simulink model "gearBoxModel_zoh"  (Simulink 6.6)
settings: Solver=FixedStepDiscrete  StartTime=0.0  StopTime=80.0  FixedStep=1  MaxStep=.001  MinStep=eps  RelTol=1e-3
undefined symbols (not defined in the file): DiscIntNeverNeededParam
settings Model: Creator=vBuskirk  LastModifiedBy=vBuskirk
settings SolverCC: ZeroCrossControl=EnableAll
settings DataIOCC: SignalLoggingName=sigsOut
settings DebuggingCC: SignalResolutionControl=TryResolveAllWithWarning  SolverPrmCheckMsg=none  MultiTaskDSMMsg=warning  MultiTaskCondExecSysMsg=none  StrictBusMsg=None
settings HardwareCC: TargetUnknown=on
settings RTWCC: IncludeERTFirstTime=on

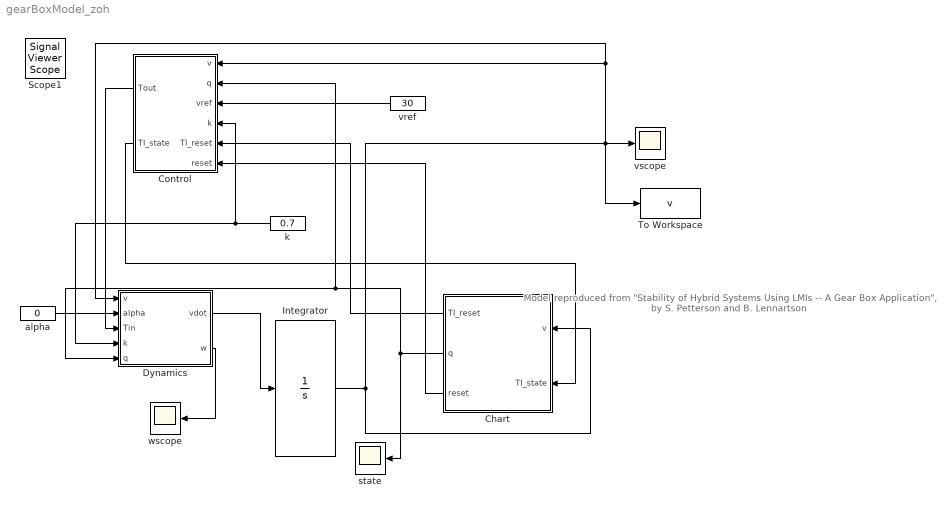
== system gearBoxModel_zoh ==
  note: Model reproduced from
      | "Stability of Hybrid Systems Using LMIs --
      | A Gear Box Application",
      | by S. Petterson and B. Lennartson
  Chart : Stateflow chart  Orientation=left
  Control : Subsystem  Orientation=left
  Dynamics : Subsystem
  Integrator : Integrator  InitialCondition=14
  To Workspace : ToWorkspace  VariableName=v  SampleTime=-1  SaveFormat=Structure
  alpha : Constant  Value=0
  k : Constant  Orientation=left  Value=0.7
  state : Scope
      settings: YMin=0  Decimation=100
  vref : Constant  Orientation=left  Value=30
  vscope : Scope
      settings: YMin=0  YMax=35  Decimation=100
  wscope : Scope
      settings: YMin=0  YMax=500  SaveName=ScopeData2  Decimation=100
  Scope1 : SignalViewerScope  IOType=viewer  RefreshTime=0.035000
  wires:
  Chart/2(q) -> state/1, Control/2(q), Dynamics/5(q)
  Dynamics/1(vdot) -> Integrator/1
  Integrator/1 -> vscope/1, Dynamics/1(v), Control/1(v), To Workspace/1, Chart/1(v)
  alpha/1 -> Dynamics/2(alpha)
  Control/1(Tout) -> Dynamics/3(Tin)
  k/1 -> Control/4(k), Dynamics/4(k)
  vref/1 -> Control/3(vref)
  Dynamics/2(w) -> wscope/1
  Chart/1(TI_reset) -> Control/5(TI_reset)
  Chart/3(reset) -> Control/6(reset)
  Control/2(TI_state) -> Chart/2(TI_state)

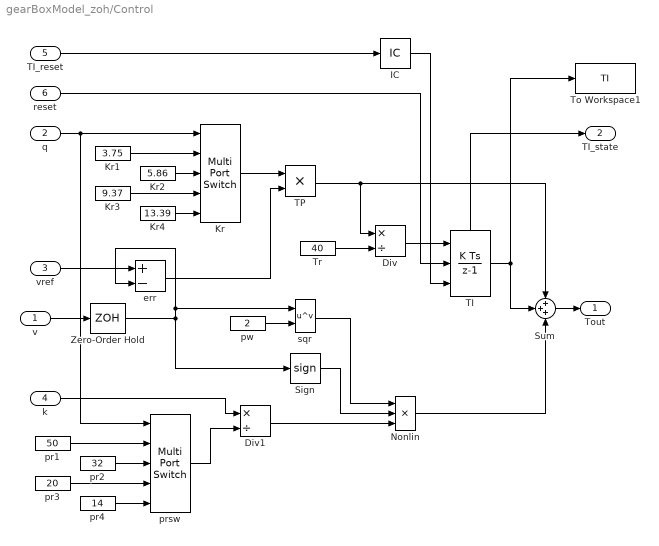
== system gearBoxModel_zoh/Control ==
  v : Inport
  q : Inport  Port=2
  vref : Inport  Port=3
  k : Inport  Port=4
  TI_reset : Inport  Port=5
  reset : Inport  Port=6
  Div : Product  Inputs=*/  OutScaling=2^-10
  Div1 : Product  Inputs=*/  OutScaling=2^-10
  IC : InitialCondition  Value=0
  Kr : MultiPortSwitch  SaturateOnIntegerOverflow=on
  Kr1 : Constant  Value=3.75
  Kr2 : Constant  Value=5.86
  Kr3 : Constant  Value=9.37
  Kr4 : Constant  Value=13.39
  Nonlin : Product  Inputs=3  RndMeth=Zero
  Sign : Signum
  Sum : Sum  Inputs=+++
  TI : DiscreteIntegrator  ExternalReset=either  InitialConditionSource=external  SampleTime=0.005  ShowStatePort=on  ICPrevOutput=DiscIntNeverNeededParam  ICPrevScaledInput=DiscIntNeverNeededParam  mask(DiscretizedDiscreteIntegrator){}
      mask init:
      | %zoh
  TP : Product  RndMeth=Zero
  To Workspace1 : ToWorkspace  VariableName=TI  SampleTime=-1  SaveFormat=Structure
  Tr : Constant  Value=40
  Zero-Order Hold : ZeroOrderHold  SampleTime=0.005
  err : Sum  Inputs=+-  OutScaling=2^-10
  pr1 : Constant  Value=50
  pr2 : Constant  Value=32
  pr3 : Constant  Value=20
  pr4 : Constant  Value=14
  prsw : MultiPortSwitch  SaturateOnIntegerOverflow=on
  pw : Constant  Value=2
  sqr : Math  Operator=pow  SaturateOnIntegerOverflow=on
  Tout : Outport
  TI_state : Outport  Port=2
  wires:
  q/1 -> Kr/1, prsw/1
  Kr1/1 -> Kr/2
  Kr2/1 -> Kr/3
  Kr3/1 -> Kr/4
  Kr4/1 -> Kr/5
  k/1 -> Div1/1
  Sum/1 -> Tout/1
  Tr/1 -> Div/2
  Kr/1 -> TP/1
  err/1 -> TP/2
  TP/1 -> Div/1, Sum/1
  pw/1 -> sqr/2
  Nonlin/1 -> Sum/3
  vref/1 -> err/1
  sqr/1 -> Nonlin/1
  Sign/1 -> Nonlin/2
  Div1/1 -> Nonlin/3
  Div/1 -> TI/1
  TI/1 -> Sum/2, To Workspace1/1
  TI_reset/1 -> IC/1
  IC/1 -> TI/3
  reset/1 -> TI/2
  TI/State -> TI_state/1
  pr1/1 -> prsw/2
  pr2/1 -> prsw/3
  pr3/1 -> prsw/4
  pr4/1 -> prsw/5
  prsw/1 -> Div1/2
  v/1 -> Zero-Order Hold/1
  Zero-Order Hold/1 -> err/2, sqr/1, Sign/1

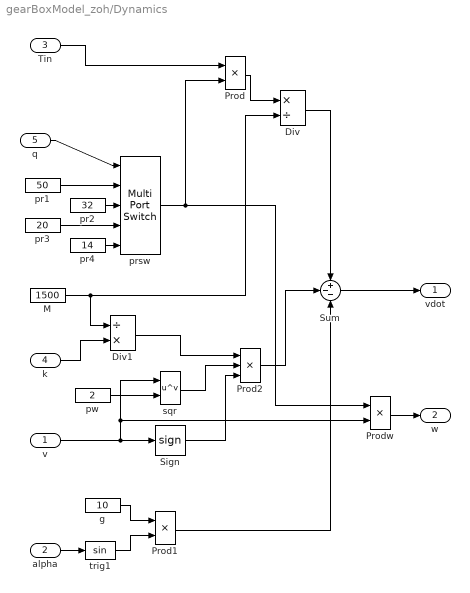
== system gearBoxModel_zoh/Dynamics ==
  v : Inport
  alpha : Inport  Port=2
  Tin : Inport  Port=3
  k : Inport  Port=4
  q : Inport  Port=5
  Div : Product  Inputs=*/  OutScaling=2^-10
  Div1 : Product  Inputs=/*  OutScaling=2^-10
  M : Constant  Value=1500
  Prod : Product  RndMeth=Zero
  Prod1 : Product  RndMeth=Zero
  Prod2 : Product  Inputs=3  RndMeth=Zero
  Prodw : Product  RndMeth=Zero
  Sign : Signum
  Sum : Sum  Inputs=+--
  g : Constant  Value=10
  pr1 : Constant  Value=50
  pr2 : Constant  Value=32
  pr3 : Constant  Value=20
  pr4 : Constant  Value=14
  prsw : MultiPortSwitch  SaturateOnIntegerOverflow=on
  pw : Constant  Value=2
  sqr : Math  Operator=pow  SaturateOnIntegerOverflow=on
  trig1 : Trigonometry
  vdot : Outport
  w : Outport  Port=2
  wires:
  alpha/1 -> trig1/1
  Prod/1 -> Div/1
  M/1 -> Div/2, Div1/1
  k/1 -> Div1/2
  Div/1 -> Sum/1
  Tin/1 -> Prod/1
  g/1 -> Prod1/1
  trig1/1 -> Prod1/2
  Prod1/1 -> Sum/3
  v/1 -> Sign/1, sqr/1, Prodw/2
  pw/1 -> sqr/2
  Div1/1 -> Prod2/1
  sqr/1 -> Prod2/2
  Sign/1 -> Prod2/3
  Prod2/1 -> Sum/2
  Prodw/1 -> w/1
  Sum/1 -> vdot/1
  q/1 -> prsw/1
  pr1/1 -> prsw/2
  pr2/1 -> prsw/3
  pr3/1 -> prsw/4
  pr4/1 -> prsw/5
  prsw/1 -> Prod/2, Prodw/1

== stateflow chart Chart ==
  state gear_4/
    entry: q=4;
  state gear_3/
    entry: q=3;
  state gear_2/
    entry: q=2;
  state gear_1/
    entry: q=1;
  gear_3 -> gear_2 [order 1] : [v <=(230/20)]/
      |     TI_reset=20 * TI_state / 32;
      |     reset;
  gear_4 -> gear_3 : [v <=(230/14)]/
      |     TI_reset=14 * TI_state / 20;
      |     reset;
  gear_2 -> gear_3 [order 2] : [v >=(500/32)]/
      |     TI_reset=32*TI_state/20;
      |     reset;
  gear_3 -> gear_4 [order 2] : [v >=(500/20)]/
      |     TI_reset=20*TI_state/14;
      |     reset;
  gear_2 -> gear_1 [order 1] : [v <=(230/32)]/
      |    TI_reset=32* TI_state / 50;
      |     reset;
  gear_1 -> gear_2 : [v >=(500/50)]/
      |     TI_reset=50 * TI_state/32;
      |      reset;
  (default) -> gear_2
  data: TI_reset output double size=1 =0; v input double size=1 =14; q output double =3; TI_state input double
  events: reset output EITHER_EDGE_EVENT
